simulink library "usask_tlm_lib"  (R2017b)
settings: Solver=ode45  StartTime=0.0  StopTime=10.0  RelTol=1e-3
undefined symbols (not defined in the file or in its folder): B, beta, d, K, L, lambda_1, m_E, m_G, mE_1, mE_2, mG_1, mG_2, nu, r1, r2, rho, T, Zc, Zc_1, Zc_2
libraries: usask_tlm_lib x6, transmission_lines x2
(part 3 of 4)

== system usask_tlm_lib/Elastic TLM Q1P2/G_1 ==
  note: Equation (17) from ven der Buhs et al. 2017
  F + P_1 : Inport
  Sum : Sum  Inputs=+------
  k = 1 : TransferFcn  Numerator=[m_G(1)*T 0]  Denominator=[T n(1)]
  k = 2 : TransferFcn  Numerator=[m_G(2)*T 0]  Denominator=[T n(2)]
  k = 3 : TransferFcn  Numerator=[m_G(3)*T 0]  Denominator=[T n(3)]
  k = 4 : TransferFcn  Numerator=[m_G(4)*T 0]  Denominator=[T n(4)]
  k = 5 : TransferFcn  Numerator=[m_G(5)*T 0]  Denominator=[T n(5)]
  k = 6 : TransferFcn  Numerator=[m_G(6)*T 0]  Denominator=[T n(6)]
  G : Outport
  wires:
  Sum/1 -> G/1
  F + P_1/1 -> k = 4/1, k = 6/1, k = 5/1, k = 1/1, Sum/1, k = 2/1, k = 3/1
  k = 3/1 -> Sum/4
  k = 1/1 -> Sum/2
  k = 2/1 -> Sum/3
  k = 4/1 -> Sum/5
  k = 5/1 -> Sum/6
  k = 6/1 -> Sum/7

== system usask_tlm_lib/Elastic TLM Q1P2/G_2 ==
  note: Equation (17) from ven der Buhs et al. 2017
  F + P_2 : Inport
  Sum : Sum  Inputs=+------
  k = 1 : TransferFcn  Numerator=[m_G(1)*T 0]  Denominator=[T n(1)]
  k = 2 : TransferFcn  Numerator=[m_G(2)*T 0]  Denominator=[T n(2)]
  k = 3 : TransferFcn  Numerator=[m_G(3)*T 0]  Denominator=[T n(3)]
  k = 4 : TransferFcn  Numerator=[m_G(4)*T 0]  Denominator=[T n(4)]
  k = 5 : TransferFcn  Numerator=[m_G(5)*T 0]  Denominator=[T n(5)]
  k = 6 : TransferFcn  Numerator=[m_G(6)*T 0]  Denominator=[T n(6)]
  G : Outport
  wires:
  Sum/1 -> G/1
  F + P_2/1 -> k = 4/1, k = 6/1, k = 5/1, k = 1/1, Sum/1, k = 2/1, k = 3/1
  k = 3/1 -> Sum/4
  k = 1/1 -> Sum/2
  k = 2/1 -> Sum/3
  k = 4/1 -> Sum/5
  k = 5/1 -> Sum/6
  k = 6/1 -> Sum/7

== system usask_tlm_lib/Elastic TLM Q1Q2/  Delay_2  ==
  G : Inport
  Transport Delay : TransportDelay  DelayTime=T_prime
  delay : Outport
  wires:
  G/1 -> Transport Delay/1
  Transport Delay/1 -> delay/1

== system usask_tlm_lib/Elastic TLM Q1Q2/Delay_1  ==
  G : Inport
  Transport Delay : TransportDelay  DelayTime=T_prime
  delay : Outport
  wires:
  G/1 -> Transport Delay/1
  Transport Delay/1 -> delay/1

== system usask_tlm_lib/Elastic TLM Q1Q2/E_1 ==
  note: Equation (14) from ven der Buhs et al. 2017
  Q_1 : Inport
  Gain : Gain  Gain=Z_c
  Sum : Sum  Inputs=++++++
  k = 1 : TransferFcn  Numerator=[m_E(1)]  Denominator=[T n(1)]
  k = 2 : TransferFcn  Numerator=[m_E(2)]  Denominator=[T n(2)]
  k = 3 : TransferFcn  Numerator=[m_E(3)]  Denominator=[T n(3)]
  k = 4 : TransferFcn  Numerator=[m_E(4)]  Denominator=[T n(4)]
  k = 5 : TransferFcn  Numerator=[m_E(5)]  Denominator=[T n(5)]
  k = 6 : TransferFcn  Numerator=[m_E(6)]  Denominator=[T n(6)]
  E : Outport
  wires:
  Gain/1 -> E/1
  Sum/1 -> Gain/1
  k = 1/1 -> Sum/1
  k = 2/1 -> Sum/2
  k = 3/1 -> Sum/3
  k = 4/1 -> Sum/4
  k = 5/1 -> Sum/5
  k = 6/1 -> Sum/6
  Q_1/1 -> k = 2/1, k = 1/1, k = 3/1, k = 6/1, k = 5/1, k = 4/1

== system usask_tlm_lib/Elastic TLM Q1Q2/E_2 ==
  note: Equation (14) from ven der Buhs et al. 2017
  Q_2 : Inport
  Gain : Gain  Gain=Z_c
  Sum : Sum  Inputs=++++++
  k = 1 : TransferFcn  Numerator=[m_E(1)]  Denominator=[T n(1)]
  k = 2 : TransferFcn  Numerator=[m_E(2)]  Denominator=[T n(2)]
  k = 3 : TransferFcn  Numerator=[m_E(3)]  Denominator=[T n(3)]
  k = 4 : TransferFcn  Numerator=[m_E(4)]  Denominator=[T n(4)]
  k = 5 : TransferFcn  Numerator=[m_E(5)]  Denominator=[T n(5)]
  k = 6 : TransferFcn  Numerator=[m_E(6)]  Denominator=[T n(6)]
  E : Outport
  wires:
  Gain/1 -> E/1
  Sum/1 -> Gain/1
  k = 1/1 -> Sum/1
  k = 2/1 -> Sum/2
  k = 3/1 -> Sum/3
  k = 4/1 -> Sum/4
  k = 5/1 -> Sum/5
  k = 6/1 -> Sum/6
  Q_2/1 -> k = 2/1, k = 1/1, k = 3/1, k = 6/1, k = 5/1, k = 4/1

== system usask_tlm_lib/Elastic TLM Q1Q2/F_1 ==
  note: Equation (15) from ven der Buhs et al. 2017
  Q_1 : Inport
  E : Inport  Port=2
  Gain : Gain  Gain=b
  Gain1 : Gain  Gain=Z_c
  Sum : Sum
  F : Outport
  wires:
  Gain/1 -> Sum/2
  Gain1/1 -> Sum/1
  Sum/1 -> F/1
  Q_1/1 -> Gain1/1
  E/1 -> Gain/1

== system usask_tlm_lib/Elastic TLM Q1Q2/F_2 ==
  note: Equation (15) from ven der Buhs et al. 2017
  E : Inport
  Q_2 : Inport  Port=2
  Gain : Gain  Gain=b
  Gain1 : Gain  Gain=Z_c
  Sum : Sum
  F : Outport
  wires:
  E/1 -> Gain/1
  Q_2/1 -> Gain1/1
  Sum/1 -> F/1
  Gain1/1 -> Sum/1
  Gain/1 -> Sum/2

== system usask_tlm_lib/Elastic TLM Q1Q2/G_1 ==
  note: Equation (17) from ven der Buhs et al. 2017
  F + P_1 : Inport
  Sum : Sum  Inputs=+------
  k = 1 : TransferFcn  Numerator=[m_G(1)*T 0]  Denominator=[T n(1)]
  k = 2 : TransferFcn  Numerator=[m_G(2)*T 0]  Denominator=[T n(2)]
  k = 3 : TransferFcn  Numerator=[m_G(3)*T 0]  Denominator=[T n(3)]
  k = 4 : TransferFcn  Numerator=[m_G(4)*T 0]  Denominator=[T n(4)]
  k = 5 : TransferFcn  Numerator=[m_G(5)*T 0]  Denominator=[T n(5)]
  k = 6 : TransferFcn  Numerator=[m_G(6)*T 0]  Denominator=[T n(6)]
  G : Outport
  wires:
  Sum/1 -> G/1
  F + P_1/1 -> k = 4/1, k = 6/1, k = 5/1, k = 1/1, Sum/1, k = 2/1, k = 3/1
  k = 3/1 -> Sum/4
  k = 1/1 -> Sum/2
  k = 2/1 -> Sum/3
  k = 4/1 -> Sum/5
  k = 5/1 -> Sum/6
  k = 6/1 -> Sum/7

== system usask_tlm_lib/Elastic TLM Q1Q2/G_2 ==
  note: Equation (17) from ven der Buhs et al. 2017
  F + P_2 : Inport
  Sum : Sum  Inputs=+------
  k = 1 : TransferFcn  Numerator=[m_G(1)*T 0]  Denominator=[T n(1)]
  k = 2 : TransferFcn  Numerator=[m_G(2)*T 0]  Denominator=[T n(2)]
  k = 3 : TransferFcn  Numerator=[m_G(3)*T 0]  Denominator=[T n(3)]
  k = 4 : TransferFcn  Numerator=[m_G(4)*T 0]  Denominator=[T n(4)]
  k = 5 : TransferFcn  Numerator=[m_G(5)*T 0]  Denominator=[T n(5)]
  k = 6 : TransferFcn  Numerator=[m_G(6)*T 0]  Denominator=[T n(6)]
  G : Outport
  wires:
  Sum/1 -> G/1
  F + P_2/1 -> k = 4/1, k = 6/1, k = 5/1, k = 1/1, Sum/1, k = 2/1, k = 3/1
  k = 3/1 -> Sum/4
  k = 1/1 -> Sum/2
  k = 2/1 -> Sum/3
  k = 4/1 -> Sum/5
  k = 5/1 -> Sum/6
  k = 6/1 -> Sum/7

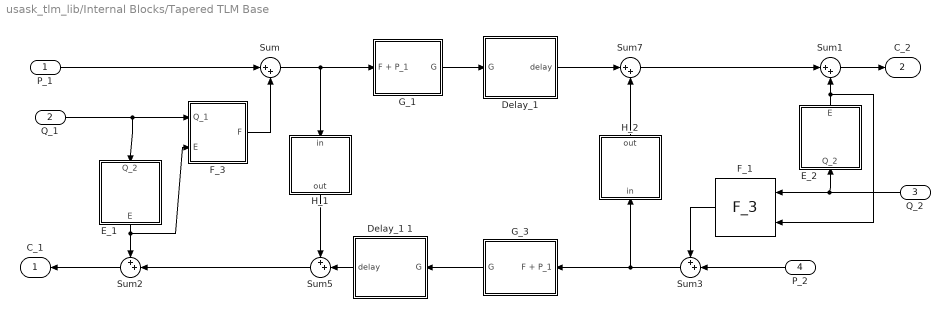
== system usask_tlm_lib/Internal Blocks/Tapered TLM Base ==
  P_1 : Inport
  Q_1 : Inport  Port=2
  Q_2 : Inport  Port=3
  P_2 : Inport  Port=4
  "Delay_1 " : Subsystem  mask{T=T_1}
      mask prompts: T "delay time"
      mask Display: disp('\fontname{Times New Roman}\ite^{-j\omegaT}', 'texmode', 'on')
  Delay_1 1 : Subsystem  mask{T=T_2}
      mask prompts: T "delay time"
      mask Display: disp('\fontname{Times New Roman}\ite^{-j\omegaT}', 'texmode', 'on')
  E_1 : Subsystem  mask{m_E=mE_1, n=n, T=T_1, Zc=Zc_1}
      mask prompts: m_E "mE"
      mask Display: disp('\fontname{Times New Roman}\fontsize{30}\itE', 'texmode', 'on')
  E_2 : Subsystem  mask{m_E=mE_2, n=n, T=T_2, Zc=Zc_2}
      mask prompts: m_E "mE"
      mask Display: disp('\fontname{Times New Roman}\fontsize{30}\itE', 'texmode', 'on')
  F_1 : usask_tlm_lib/Internal Blocks/Tapered TLM Base/F_3  Zc=Zc_2  b=b_2  F_k=F_k2
      settings: SourceProductName=USask Transmission Line Model Library
  F_3 : Subsystem  mask{Zc=Zc_1, b=b_1, F_k=F_k1}
      mask prompts: F_k "Scale"
      mask Display: disp('\fontname{Times New Roman}\fontsize{30}\itF', 'texmode', 'on')
  G_1 : Subsystem  mask{m_G=mG_1, n=n, T=T_1, H_DC=H_2DC}
      mask prompts: m_G "mG"
      mask Display: disp('\fontname{Times New Roman}\fontsize{30}\itG', 'texmode', 'on')
  G_3 : Subsystem  mask{m_G=mG_2, n=n, T=T_2, H_DC=H_1DC}
      mask prompts: m_G "mG"
      mask Display: disp('\fontname{Times New Roman}\fontsize{30}\itG', 'texmode', 'on')
  H_1 : Subsystem  mask{H_a=H_1a, H_b=H_1b, T=T_1+T_2}
      mask prompts: T "T (round trip)"
      mask Display: disp('\fontname{Times New Roman}\fontsize{30}\itH', 'texmode', 'on')
  H_2 : Subsystem  mask{H_a=H_2a, H_b=H_2b, T=T_1+T_2}
      mask prompts: T "T (round trip)"
      mask Display: disp('\fontname{Times New Roman}\fontsize{30}\itH', 'texmode', 'on')
  Sum : Sum  Inputs=|++
  Sum1 : Sum  Inputs=|++
  Sum2 : Sum  Inputs=++|
  Sum3 : Sum  Inputs=++|
  Sum5 : Sum  Inputs=++|
  Sum7 : Sum  Inputs=|++
  C_1 : Outport
  " C_2" : Outport  Port=2
  wires:
  F_1/1 -> Sum3/1
  Sum5/1 -> Sum2/2
  F_3/1(F) -> Sum/2
  P_2/1 -> Sum3/2
  E_2/1(E) -> F_1/2, Sum1/2
  G_1/1(G) -> "Delay_1 "/1(G)
  Q_2/1 -> F_1/1, E_2/1(Q_2)
  Q_1/1 -> F_3/1(Q_1), E_1/1(Q_2)
  Sum1/1 -> " C_2"/1
  Sum3/1 -> G_3/1(F + P_1), H_2/1(in)
  Sum7/1 -> Sum1/1
  H_2/1(out) -> Sum7/2
  Delay_1 1/1(delay) -> Sum5/2
  E_1/1(E) -> F_3/2(E), Sum2/1
  Sum2/1 -> C_1/1
  Sum/1 -> H_1/1(in), G_1/1(F + P_1)
  P_1/1 -> Sum/1
  H_1/1(out) -> Sum5/1
  G_3/1(G) -> Delay_1 1/1(G)
  "Delay_1 "/1(delay) -> Sum7/1

== system usask_tlm_lib/Internal Blocks/Tapered TLM Segment ==
  C_1in : Inport
  C_2in : Inport  Port=2
  Add : Sum
  Add1 : Sum
  Add2 : Sum  Inputs=+-
  Add3 : Sum  Inputs=+-
  Gain{,1..2,4} (4 alike) : Gain  Gain=1/2
  Gain3 : Gain  Gain=1/Zc_1
  Gain5 : Gain  Gain=1/Zc_2
  Tapered TLM Base : usask_tlm_lib/Internal Blocks/Tapered TLM Base  Zc_1=Zc_1  Zc_2=Zc_2  beta=beta  T=T  lambda_1=lambda_1
      settings: SourceProductName=USask Transmission Line Model Library
  " C_1out" : Outport
  " C_2out" : Outport  Port=2
  wires:
  C_1in/1 -> Add/2, Add2/1
  Tapered TLM Base/1 -> " C_1out"/1, Add/1, Add2/2
  Add/1 -> Gain/1
  Gain/1 -> Tapered TLM Base/1
  Gain1/1 -> Tapered TLM Base/4
  Add1/1 -> Gain1/1
  Tapered TLM Base/2 -> " C_2out"/1, Add3/2, Add1/2
  Add2/1 -> Gain2/1
  Gain2/1 -> Gain3/1
  Gain3/1 -> Tapered TLM Base/2
  Gain4/1 -> Gain5/1
  Add3/1 -> Gain4/1
  Gain5/1 -> Tapered TLM Base/3
  C_2in/1 -> Add3/1, Add1/1

== system usask_tlm_lib/TLM Johnston P1P2/E2 ==
  In : Inport
  Transfer Fcn : TransferFcn  Numerator=[R]  Denominator=[K*T 1]
  Out : Outport
  wires:
  Transfer Fcn/1 -> Out/1
  In/1 -> Transfer Fcn/1

== system usask_tlm_lib/TLM Johnston P1P2/F2 ==
  In : Inport
  Gain : Gain  Gain=Zc
  Out : Outport
  wires:
  Gain/1 -> Out/1
  In/1 -> Gain/1

== system usask_tlm_lib/TLM Johnston P1P2/G1 ==
  In : Inport
  G2 : Subsystem  mask(Johnston G2){modelNumber=modelNumber}
      mask prompts: modelNumber "Model"
      mask help: This implements Johnston's G2 models. Model may be 1, 2 or 3 (see paper). Model 1 may be unstable for large beta.
      mask init:
      | k=4;%this must match order of diagram
      | m=nan(k,1);
      | m(1)=2.2457;
      | if k>1
      | m(2)=6.8400;
      | end
      | for i=3:k
      |     m(i)=3*m(i-1);
      | end
      | 
      | 
      | n=nan(k,1);
      | n(1)=42.849;
      | for i=2:k
      |     n(i)=9*n(i-1);
      | end
      | 
      | 
      | if modelNumber==1
      |         bypass1=false;
      |         bypass2=true;
      |         numGain=2;%numerator gain
      | elseif modelNumber==2
      |     bypass1=true;
      |         bypass2=false;
      |         numGain=2;%numerator gain
      | elseif modelNumber==3
      |         bypass1=false;
      |         bypass2=false;
      |         numGain=1;%numerator gain
      | else
      |     warning('Model number must be 1, 2, or 3')
      | end
  Transfer Fcn : TransferFcn  Numerator=[K*beta*r^2/nu*exp(-4*beta) 1]  Denominator=[K*beta*r^2/nu 1]
  Out : Outport
  wires:
  In/1 -> Transfer Fcn/1
  Transfer Fcn/1 -> G2/1(In)
  G2/1(Out) -> Out/1

== system usask_tlm_lib/TLM Johnston P1P2/G2 ==
  In : Inport
  G2 : Subsystem  mask(Johnston G2){modelNumber=modelNumber}
      mask prompts: modelNumber "Model"
      mask help: This implements Johnston's G2 models. Model may be 1, 2 or 3 (see paper). Model 1 may be unstable for large beta.
      mask init: same as usask_tlm_lib/TLM Johnston P1P2/G1/G2
  Transfer Fcn : TransferFcn  Numerator=[K*beta*r^2/nu*exp(-4*beta) 1]  Denominator=[K*beta*r^2/nu 1]
  Out : Outport
  wires:
  In/1 -> Transfer Fcn/1
  Transfer Fcn/1 -> G2/1(In)
  G2/1(Out) -> Out/1

== system usask_tlm_lib/TLM Johnston P1Q2/Ea ==
  In : Inport
  Transfer Fcn : TransferFcn  Numerator=[R]  Denominator=[K*T 1]
  Out : Outport
  wires:
  In/1 -> Transfer Fcn/1
  Transfer Fcn/1 -> Out/1

== system usask_tlm_lib/TLM Johnston P1Q2/Eb ==
  In : Inport
  Transfer Fcn : TransferFcn  Numerator=[R]  Denominator=[K*T 1]
  Out : Outport
  wires:
  In/1 -> Transfer Fcn/1
  Transfer Fcn/1 -> Out/1

== system usask_tlm_lib/TLM Johnston P1Q2/Fa ==
  In : Inport
  Gain : Gain  Gain=Zc
  Out : Outport
  wires:
  In/1 -> Gain/1
  Gain/1 -> Out/1

== system usask_tlm_lib/TLM Johnston P1Q2/Fb ==
  In : Inport
  Gain : Gain  Gain=Zc
  Out : Outport
  wires:
  In/1 -> Gain/1
  Gain/1 -> Out/1

== system usask_tlm_lib/TLM Johnston P1Q2/Ga ==
  In : Inport
  G2 : Subsystem  mask(Johnston G2){modelNumber=modelNumber}
      mask prompts: modelNumber "Model"
      mask help: This implements Johnston's G2 models. Model may be 1, 2 or 3 (see paper). Model 1 may be unstable for large beta.
      mask init: same as usask_tlm_lib/TLM Johnston P1P2/G1/G2
  Transfer Fcn : TransferFcn  Numerator=[K*beta*r^2/nu*exp(-4*beta) 1]  Denominator=[K*beta*r^2/nu 1]
  Out : Outport
  wires:
  G2/1(Out) -> Out/1
  Transfer Fcn/1 -> G2/1(In)
  In/1 -> Transfer Fcn/1

== system usask_tlm_lib/TLM Johnston P1Q2/Gb ==
  In : Inport
  G2 : Subsystem  mask(Johnston G2){modelNumber=modelNumber}
      mask prompts: modelNumber "Model"
      mask help: This implements Johnston's G2 models. Model may be 1, 2 or 3 (see paper). Model 1 may be unstable for large beta.
      mask init: same as usask_tlm_lib/TLM Johnston P1P2/G1/G2
  Transfer Fcn : TransferFcn  Numerator=[K*beta*r^2/nu*exp(-4*beta) 1]  Denominator=[K*beta*r^2/nu 1]
  Out : Outport
  wires:
  G2/1(Out) -> Out/1
  Transfer Fcn/1 -> G2/1(In)
  In/1 -> Transfer Fcn/1

== system usask_tlm_lib/TLM Johnston Q1P2/Ea ==
  In : Inport
  Transfer Fcn : TransferFcn  Numerator=[R]  Denominator=[K*T 1]
  Out : Outport
  wires:
  In/1 -> Transfer Fcn/1
  Transfer Fcn/1 -> Out/1

== system usask_tlm_lib/TLM Johnston Q1P2/Eb ==
  In : Inport
  Transfer Fcn : TransferFcn  Numerator=[R]  Denominator=[K*T 1]
  Out : Outport
  wires:
  In/1 -> Transfer Fcn/1
  Transfer Fcn/1 -> Out/1

== system usask_tlm_lib/TLM Johnston Q1P2/Fa ==
  In : Inport
  Gain : Gain  Gain=Zc
  Out : Outport
  wires:
  In/1 -> Gain/1
  Gain/1 -> Out/1

== system usask_tlm_lib/TLM Johnston Q1P2/Fb ==
  In : Inport
  Gain : Gain  Gain=Zc
  Out : Outport
  wires:
  In/1 -> Gain/1
  Gain/1 -> Out/1

== system usask_tlm_lib/TLM Johnston Q1P2/Ga ==
  In : Inport
  G2 : Subsystem  mask(Johnston G2){modelNumber=modelNumber}
      mask prompts: modelNumber "Model"
      mask help: This implements Johnston's G2 models. Model may be 1, 2 or 3 (see paper). Model 1 may be unstable for large beta.
      mask init: same as usask_tlm_lib/TLM Johnston P1P2/G1/G2
  Transfer Fcn : TransferFcn  Numerator=[K*beta*r^2/nu*exp(-4*beta) 1]  Denominator=[K*beta*r^2/nu 1]
  Out : Outport
  wires:
  G2/1(Out) -> Out/1
  Transfer Fcn/1 -> G2/1(In)
  In/1 -> Transfer Fcn/1

== system usask_tlm_lib/TLM Johnston Q1P2/Gb ==
  In : Inport
  G2 : Subsystem  mask(Johnston G2){modelNumber=modelNumber}
      mask prompts: modelNumber "Model"
      mask help: This implements Johnston's G2 models. Model may be 1, 2 or 3 (see paper). Model 1 may be unstable for large beta.
      mask init: same as usask_tlm_lib/TLM Johnston P1P2/G1/G2
  Transfer Fcn : TransferFcn  Numerator=[K*beta*r^2/nu*exp(-4*beta) 1]  Denominator=[K*beta*r^2/nu 1]
  Out : Outport
  wires:
  G2/1(Out) -> Out/1
  Transfer Fcn/1 -> G2/1(In)
  In/1 -> Transfer Fcn/1

== system usask_tlm_lib/TLM Johnston Q1Q2/Ea ==
  In : Inport
  Transfer Fcn : TransferFcn  Numerator=[R]  Denominator=[K*T 1]
  Out : Outport
  wires:
  In/1 -> Transfer Fcn/1
  Transfer Fcn/1 -> Out/1

== system usask_tlm_lib/TLM Johnston Q1Q2/Eb ==
  In : Inport
  Transfer Fcn : TransferFcn  Numerator=[R]  Denominator=[K*T 1]
  Out : Outport
  wires:
  In/1 -> Transfer Fcn/1
  Transfer Fcn/1 -> Out/1

== system usask_tlm_lib/TLM Johnston Q1Q2/Fa ==
  In : Inport
  Gain : Gain  Gain=Zc
  Out : Outport
  wires:
  In/1 -> Gain/1
  Gain/1 -> Out/1

== system usask_tlm_lib/TLM Johnston Q1Q2/Fb ==
  In : Inport
  Gain : Gain  Gain=Zc
  Out : Outport
  wires:
  In/1 -> Gain/1
  Gain/1 -> Out/1

== system usask_tlm_lib/TLM Johnston Q1Q2/Ga ==
  In : Inport
  G2 : Subsystem  mask(Johnston G2){modelNumber=modelNumber}
      mask prompts: modelNumber "Model"
      mask help: This implements Johnston's G2 models. Model may be 1, 2 or 3 (see paper). Model 1 may be unstable for large beta.
      mask init: same as usask_tlm_lib/TLM Johnston P1P2/G1/G2
  Transfer Fcn : TransferFcn  Numerator=[K*beta*r^2/nu*exp(-4*beta) 1]  Denominator=[K*beta*r^2/nu 1]
  Out : Outport
  wires:
  G2/1(Out) -> Out/1
  Transfer Fcn/1 -> G2/1(In)
  In/1 -> Transfer Fcn/1

== system usask_tlm_lib/TLM Johnston Q1Q2/Gb ==
  In : Inport
  G2 : Subsystem  mask(Johnston G2){modelNumber=modelNumber}
      mask prompts: modelNumber "Model"
      mask help: This implements Johnston's G2 models. Model may be 1, 2 or 3 (see paper). Model 1 may be unstable for large beta.
      mask init: same as usask_tlm_lib/TLM Johnston P1P2/G1/G2
  Transfer Fcn : TransferFcn  Numerator=[K*beta*r^2/nu*exp(-4*beta) 1]  Denominator=[K*beta*r^2/nu 1]
  Out : Outport
  wires:
  G2/1(Out) -> Out/1
  Transfer Fcn/1 -> G2/1(In)
  In/1 -> Transfer Fcn/1

== system usask_tlm_lib/TLM Krus P1P2/E1 ==
  In : Inport
  Transfer Fcn : TransferFcn  Numerator=[R]  Denominator=[K*T 1]
  Out : Outport
  wires:
  Transfer Fcn/1 -> Out/1
  In/1 -> Transfer Fcn/1

== system usask_tlm_lib/TLM Krus P1P2/E2 ==
  In : Inport
  Transfer Fcn : TransferFcn  Numerator=[R]  Denominator=[K*T 1]
  Out : Outport
  wires:
  Transfer Fcn/1 -> Out/1
  In/1 -> Transfer Fcn/1

== system usask_tlm_lib/TLM Krus P1P2/F1 ==
  In : Inport
  Gain : Gain  Gain=Zc
  Out : Outport
  wires:
  Gain/1 -> Out/1
  In/1 -> Gain/1

== system usask_tlm_lib/TLM Krus P1P2/F2 ==
  In : Inport
  Gain : Gain  Gain=Zc
  Out : Outport
  wires:
  Gain/1 -> Out/1
  In/1 -> Gain/1

== system usask_tlm_lib/TLM Krus P1P2/G1 ==
  In : Inport
  Transfer Fcn : TransferFcn  Numerator=[K*T*exp(-R*A/(2*rho*c)) 1]  Denominator=[K*T 1]
  Out : Outport
  wires:
  Transfer Fcn/1 -> Out/1
  In/1 -> Transfer Fcn/1

== system usask_tlm_lib/TLM Krus P1P2/G2 ==
  In : Inport
  Transfer Fcn : TransferFcn  Numerator=[K*T*exp(-R*A/(2*rho*c)) 1]  Denominator=[K*T 1]
  Out : Outport
  wires:
  Transfer Fcn/1 -> Out/1
  In/1 -> Transfer Fcn/1

== system usask_tlm_lib/TLM Krus P1Q2/E1 ==
  In : Inport
  Transfer Fcn : TransferFcn  Numerator=[R]  Denominator=[K*T 1]
  Out : Outport
  wires:
  In/1 -> Transfer Fcn/1
  Transfer Fcn/1 -> Out/1

== system usask_tlm_lib/TLM Krus P1Q2/E2 ==
  In : Inport
  Transfer Fcn : TransferFcn  Numerator=[R]  Denominator=[K*T 1]
  Out : Outport
  wires:
  In/1 -> Transfer Fcn/1
  Transfer Fcn/1 -> Out/1

== system usask_tlm_lib/TLM Krus P1Q2/F1 ==
  In : Inport
  Gain : Gain  Gain=Zc
  Out : Outport
  wires:
  In/1 -> Gain/1
  Gain/1 -> Out/1

== system usask_tlm_lib/TLM Krus P1Q2/F2 ==
  In : Inport
  Gain : Gain  Gain=Zc
  Out : Outport
  wires:
  In/1 -> Gain/1
  Gain/1 -> Out/1

== system usask_tlm_lib/TLM Krus P1Q2/G1 ==
  In : Inport
  Transfer Fcn : TransferFcn  Numerator=[K*T*exp(-R*A/(2*rho*c)) 1]  Denominator=[K*T 1]
  Out : Outport
  wires:
  In/1 -> Transfer Fcn/1
  Transfer Fcn/1 -> Out/1

== system usask_tlm_lib/TLM Krus P1Q2/G2 ==
  In : Inport
  Transfer Fcn : TransferFcn  Numerator=[K*T*exp(-R*A/(2*rho*c)) 1]  Denominator=[K*T 1]
  Out : Outport
  wires:
  In/1 -> Transfer Fcn/1
  Transfer Fcn/1 -> Out/1

== system usask_tlm_lib/TLM Krus Q1P2/E1 ==
  In : Inport
  Transfer Fcn : TransferFcn  Numerator=[R]  Denominator=[K*T 1]
  Out : Outport
  wires:
  Transfer Fcn/1 -> Out/1
  In/1 -> Transfer Fcn/1

== system usask_tlm_lib/TLM Krus Q1P2/E2 ==
  In : Inport
  Transfer Fcn : TransferFcn  Numerator=[R]  Denominator=[K*T 1]
  Out : Outport
  wires:
  Transfer Fcn/1 -> Out/1
  In/1 -> Transfer Fcn/1

== system usask_tlm_lib/TLM Krus Q1P2/F1 ==
  In : Inport
  Gain : Gain  Gain=Zc
  Out : Outport
  wires:
  Gain/1 -> Out/1
  In/1 -> Gain/1

== system usask_tlm_lib/TLM Krus Q1P2/F2 ==
  In : Inport
  Gain : Gain  Gain=Zc
  Out : Outport
  wires:
  Gain/1 -> Out/1
  In/1 -> Gain/1

== system usask_tlm_lib/TLM Krus Q1P2/G1 ==
  In : Inport
  Transfer Fcn : TransferFcn  Numerator=[K*T*exp(-R*A/(2*rho*c)) 1]  Denominator=[K*T 1]
  Out : Outport
  wires:
  Transfer Fcn/1 -> Out/1
  In/1 -> Transfer Fcn/1

== system usask_tlm_lib/TLM Krus Q1P2/G2 ==
  In : Inport
  Transfer Fcn : TransferFcn  Numerator=[K*T*exp(-R*A/(2*rho*c)) 1]  Denominator=[K*T 1]
  Out : Outport
  wires:
  Transfer Fcn/1 -> Out/1
  In/1 -> Transfer Fcn/1

== system usask_tlm_lib/TLM Krus Q1Q2/E1 ==
  In : Inport
  Transfer Fcn : TransferFcn  Numerator=[R]  Denominator=[K*T 1]
  Out : Outport
  wires:
  Transfer Fcn/1 -> Out/1
  In/1 -> Transfer Fcn/1

== system usask_tlm_lib/TLM Krus Q1Q2/E2 ==
  In : Inport
  Transfer Fcn : TransferFcn  Numerator=[R]  Denominator=[K*T 1]
  Out : Outport
  wires:
  Transfer Fcn/1 -> Out/1
  In/1 -> Transfer Fcn/1

== system usask_tlm_lib/TLM Krus Q1Q2/F1 ==
  In : Inport
  Gain : Gain  Gain=Zc
  Out : Outport
  wires:
  Gain/1 -> Out/1
  In/1 -> Gain/1

== system usask_tlm_lib/TLM Krus Q1Q2/F2 ==
  In : Inport
  Gain : Gain  Gain=Zc
  Out : Outport
  wires:
  Gain/1 -> Out/1
  In/1 -> Gain/1

== system usask_tlm_lib/TLM Krus Q1Q2/G1 ==
  In : Inport
  Transfer Fcn : TransferFcn  Numerator=[K*T*exp(-R*A/(2*rho*c)) 1]  Denominator=[K*T 1]
  Out : Outport
  wires:
  Transfer Fcn/1 -> Out/1
  In/1 -> Transfer Fcn/1

== system usask_tlm_lib/TLM Krus Q1Q2/G2 ==
  In : Inport
  Transfer Fcn : TransferFcn  Numerator=[K*T*exp(-R*A/(2*rho*c)) 1]  Denominator=[K*T 1]
  Out : Outport
  wires:
  Transfer Fcn/1 -> Out/1
  In/1 -> Transfer Fcn/1

== system usask_tlm_lib/Tapered Elastic TLM P1P2/  Delay_2  ==
  G : Inport
  Transport Delay : TransportDelay  DelayTime=T_prime
  delay : Outport
  wires:
  G/1 -> Transport Delay/1
  Transport Delay/1 -> delay/1

== system usask_tlm_lib/Tapered Elastic TLM P1P2/Delay_1  ==
  G : Inport
  Transport Delay : TransportDelay  DelayTime=T_prime
  delay : Outport
  wires:
  G/1 -> Transport Delay/1
  Transport Delay/1 -> delay/1

== system usask_tlm_lib/Tapered Elastic TLM P1P2/E_1 ==
  note: Equation (14) from ven der Buhs et al. 2017
  Q_1 : Inport
  Gain : Gain  Gain=Z_c
  Sum : Sum  Inputs=++++++
  k = 1 : TransferFcn  Numerator=[m_E(1)]  Denominator=[T n(1)]
  k = 2 : TransferFcn  Numerator=[m_E(2)]  Denominator=[T n(2)]
  k = 3 : TransferFcn  Numerator=[m_E(3)]  Denominator=[T n(3)]
  k = 4 : TransferFcn  Numerator=[m_E(4)]  Denominator=[T n(4)]
  k = 5 : TransferFcn  Numerator=[m_E(5)]  Denominator=[T n(5)]
  k = 6 : TransferFcn  Numerator=[m_E(6)]  Denominator=[T n(6)]
  E : Outport
  wires:
  Gain/1 -> E/1
  Sum/1 -> Gain/1
  k = 1/1 -> Sum/1
  k = 2/1 -> Sum/2
  k = 3/1 -> Sum/3
  k = 4/1 -> Sum/4
  k = 5/1 -> Sum/5
  k = 6/1 -> Sum/6
  Q_1/1 -> k = 2/1, k = 1/1, k = 3/1, k = 6/1, k = 5/1, k = 4/1

== system usask_tlm_lib/Tapered Elastic TLM P1P2/E_2 ==
  note: Equation (14) from ven der Buhs et al. 2017
  Q_2 : Inport
  Gain : Gain  Gain=Z_c
  Sum : Sum  Inputs=++++++
  k = 1 : TransferFcn  Numerator=[m_E(1)]  Denominator=[T n(1)]
  k = 2 : TransferFcn  Numerator=[m_E(2)]  Denominator=[T n(2)]
  k = 3 : TransferFcn  Numerator=[m_E(3)]  Denominator=[T n(3)]
  k = 4 : TransferFcn  Numerator=[m_E(4)]  Denominator=[T n(4)]
  k = 5 : TransferFcn  Numerator=[m_E(5)]  Denominator=[T n(5)]
  k = 6 : TransferFcn  Numerator=[m_E(6)]  Denominator=[T n(6)]
  E : Outport
  wires:
  Gain/1 -> E/1
  Sum/1 -> Gain/1
  k = 1/1 -> Sum/1
  k = 2/1 -> Sum/2
  k = 3/1 -> Sum/3
  k = 4/1 -> Sum/4
  k = 5/1 -> Sum/5
  k = 6/1 -> Sum/6
  Q_2/1 -> k = 2/1, k = 1/1, k = 3/1, k = 6/1, k = 5/1, k = 4/1

== system usask_tlm_lib/Tapered Elastic TLM P1P2/F_1 ==
  note: Equation (15) from ven der Buhs et al. 2017
  Q_1 : Inport
  E : Inport  Port=2
  Gain : Gain  Gain=b
  Gain1 : Gain  Gain=Z_c
  Sum : Sum
  Out1 : Outport
  wires:
  Gain/1 -> Sum/2
  Gain1/1 -> Sum/1
  Sum/1 -> Out1/1
  Q_1/1 -> Gain1/1
  E/1 -> Gain/1

== system usask_tlm_lib/Tapered Elastic TLM P1P2/F_2 ==
  note: Equation (15) from ven der Buhs et al. 2017
  E : Inport
  Q_2 : Inport  Port=2
  Gain : Gain  Gain=b
  Gain1 : Gain  Gain=Z_c
  Sum : Sum
  F : Outport
  wires:
  E/1 -> Gain/1
  Q_2/1 -> Gain1/1
  Sum/1 -> F/1
  Gain1/1 -> Sum/1
  Gain/1 -> Sum/2

== system usask_tlm_lib/Tapered Elastic TLM P1P2/G_1 ==
  note: Equation (17) from ven der Buhs et al. 2017
  F + P_1 : Inport
  Sum : Sum  Inputs=+------
  k = 1 : TransferFcn  Numerator=[m_G(1)*T 0]  Denominator=[T n(1)]
  k = 2 : TransferFcn  Numerator=[m_G(2)*T 0]  Denominator=[T n(2)]
  k = 3 : TransferFcn  Numerator=[m_G(3)*T 0]  Denominator=[T n(3)]
  k = 4 : TransferFcn  Numerator=[m_G(4)*T 0]  Denominator=[T n(4)]
  k = 5 : TransferFcn  Numerator=[m_G(5)*T 0]  Denominator=[T n(5)]
  k = 6 : TransferFcn  Numerator=[m_G(6)*T 0]  Denominator=[T n(6)]
  G : Outport
  wires:
  Sum/1 -> G/1
  F + P_1/1 -> k = 4/1, k = 6/1, k = 5/1, k = 1/1, Sum/1, k = 2/1, k = 3/1
  k = 3/1 -> Sum/4
  k = 1/1 -> Sum/2
  k = 2/1 -> Sum/3
  k = 4/1 -> Sum/5
  k = 5/1 -> Sum/6
  k = 6/1 -> Sum/7

== system usask_tlm_lib/Tapered Elastic TLM P1P2/G_2 ==
  note: Equation (17) from ven der Buhs et al. 2017
  F + P_2 : Inport
  Sum : Sum  Inputs=+------
  k = 1 : TransferFcn  Numerator=[m_G(1)*T 0]  Denominator=[T n(1)]
  k = 2 : TransferFcn  Numerator=[m_G(2)*T 0]  Denominator=[T n(2)]
  k = 3 : TransferFcn  Numerator=[m_G(3)*T 0]  Denominator=[T n(3)]
  k = 4 : TransferFcn  Numerator=[m_G(4)*T 0]  Denominator=[T n(4)]
  k = 5 : TransferFcn  Numerator=[m_G(5)*T 0]  Denominator=[T n(5)]
  k = 6 : TransferFcn  Numerator=[m_G(6)*T 0]  Denominator=[T n(6)]
  G : Outport
  wires:
  Sum/1 -> G/1
  F + P_2/1 -> k = 4/1, k = 6/1, k = 5/1, k = 1/1, Sum/1, k = 2/1, k = 3/1
  k = 3/1 -> Sum/4
  k = 1/1 -> Sum/2
  k = 2/1 -> Sum/3
  k = 4/1 -> Sum/5
  k = 5/1 -> Sum/6
  k = 6/1 -> Sum/7

== system usask_tlm_lib/Tapered Elastic TLM P1Q2/  Delay_2  ==
  G : Inport
  Transport Delay : TransportDelay  DelayTime=T_prime
  delay : Outport
  wires:
  G/1 -> Transport Delay/1
  Transport Delay/1 -> delay/1

== system usask_tlm_lib/Tapered Elastic TLM P1Q2/Delay_1  ==
  G : Inport
  Transport Delay : TransportDelay  DelayTime=T_prime
  delay : Outport
  wires:
  G/1 -> Transport Delay/1
  Transport Delay/1 -> delay/1

== system usask_tlm_lib/Tapered Elastic TLM P1Q2/E_1 ==
  note: Equation (14) from ven der Buhs et al. 2017
  Q_1 : Inport
  Gain : Gain  Gain=Z_c
  Sum : Sum  Inputs=++++++
  k = 1 : TransferFcn  Numerator=[m_E(1)]  Denominator=[T n(1)]
  k = 2 : TransferFcn  Numerator=[m_E(2)]  Denominator=[T n(2)]
  k = 3 : TransferFcn  Numerator=[m_E(3)]  Denominator=[T n(3)]
  k = 4 : TransferFcn  Numerator=[m_E(4)]  Denominator=[T n(4)]
  k = 5 : TransferFcn  Numerator=[m_E(5)]  Denominator=[T n(5)]
  k = 6 : TransferFcn  Numerator=[m_E(6)]  Denominator=[T n(6)]
  E : Outport
  wires:
  Gain/1 -> E/1
  Sum/1 -> Gain/1
  k = 1/1 -> Sum/1
  k = 2/1 -> Sum/2
  k = 3/1 -> Sum/3
  k = 4/1 -> Sum/4
  k = 5/1 -> Sum/5
  k = 6/1 -> Sum/6
  Q_1/1 -> k = 2/1, k = 1/1, k = 3/1, k = 6/1, k = 5/1, k = 4/1

== system usask_tlm_lib/Tapered Elastic TLM P1Q2/E_2 ==
  note: Equation (14) from ven der Buhs et al. 2017
  Q_2 : Inport
  Gain : Gain  Gain=Z_c
  Sum : Sum  Inputs=++++++
  k = 1 : TransferFcn  Numerator=[m_E(1)]  Denominator=[T n(1)]
  k = 2 : TransferFcn  Numerator=[m_E(2)]  Denominator=[T n(2)]
  k = 3 : TransferFcn  Numerator=[m_E(3)]  Denominator=[T n(3)]
  k = 4 : TransferFcn  Numerator=[m_E(4)]  Denominator=[T n(4)]
  k = 5 : TransferFcn  Numerator=[m_E(5)]  Denominator=[T n(5)]
  k = 6 : TransferFcn  Numerator=[m_E(6)]  Denominator=[T n(6)]
  E : Outport
  wires:
  Gain/1 -> E/1
  Sum/1 -> Gain/1
  k = 1/1 -> Sum/1
  k = 2/1 -> Sum/2
  k = 3/1 -> Sum/3
  k = 4/1 -> Sum/4
  k = 5/1 -> Sum/5
  k = 6/1 -> Sum/6
  Q_2/1 -> k = 2/1, k = 1/1, k = 3/1, k = 6/1, k = 5/1, k = 4/1

== system usask_tlm_lib/Tapered Elastic TLM P1Q2/F_1 ==
  note: Equation (15) from ven der Buhs et al. 2017
  Q_1 : Inport
  E : Inport  Port=2
  Gain : Gain  Gain=b
  Gain1 : Gain  Gain=Z_c
  Sum : Sum
  F : Outport
  wires:
  Gain/1 -> Sum/2
  Gain1/1 -> Sum/1
  Sum/1 -> F/1
  Q_1/1 -> Gain1/1
  E/1 -> Gain/1

== system usask_tlm_lib/Tapered Elastic TLM P1Q2/F_2 ==
  note: Equation (15) from ven der Buhs et al. 2017
  E : Inport
  Q_2 : Inport  Port=2
  Gain : Gain  Gain=b
  Gain1 : Gain  Gain=Z_c
  Sum : Sum
  Out1 : Outport
  wires:
  E/1 -> Gain/1
  Q_2/1 -> Gain1/1
  Sum/1 -> Out1/1
  Gain1/1 -> Sum/1
  Gain/1 -> Sum/2

== system usask_tlm_lib/Tapered Elastic TLM P1Q2/G_1 ==
  note: Equation (17) from ven der Buhs et al. 2017
  F + P_1 : Inport
  Sum : Sum  Inputs=+------
  k = 1 : TransferFcn  Numerator=[m_G(1)*T 0]  Denominator=[T n(1)]
  k = 2 : TransferFcn  Numerator=[m_G(2)*T 0]  Denominator=[T n(2)]
  k = 3 : TransferFcn  Numerator=[m_G(3)*T 0]  Denominator=[T n(3)]
  k = 4 : TransferFcn  Numerator=[m_G(4)*T 0]  Denominator=[T n(4)]
  k = 5 : TransferFcn  Numerator=[m_G(5)*T 0]  Denominator=[T n(5)]
  k = 6 : TransferFcn  Numerator=[m_G(6)*T 0]  Denominator=[T n(6)]
  G : Outport
  wires:
  Sum/1 -> G/1
  F + P_1/1 -> k = 4/1, k = 6/1, k = 5/1, k = 1/1, Sum/1, k = 2/1, k = 3/1
  k = 3/1 -> Sum/4
  k = 1/1 -> Sum/2
  k = 2/1 -> Sum/3
  k = 4/1 -> Sum/5
  k = 5/1 -> Sum/6
  k = 6/1 -> Sum/7

== system usask_tlm_lib/Tapered Elastic TLM P1Q2/G_2 ==
  note: Equation (17) from ven der Buhs et al. 2017
  F + P_2 : Inport
  Sum : Sum  Inputs=+------
  k = 1 : TransferFcn  Numerator=[m_G(1)*T 0]  Denominator=[T n(1)]
  k = 2 : TransferFcn  Numerator=[m_G(2)*T 0]  Denominator=[T n(2)]
  k = 3 : TransferFcn  Numerator=[m_G(3)*T 0]  Denominator=[T n(3)]
  k = 4 : TransferFcn  Numerator=[m_G(4)*T 0]  Denominator=[T n(4)]
  k = 5 : TransferFcn  Numerator=[m_G(5)*T 0]  Denominator=[T n(5)]
  k = 6 : TransferFcn  Numerator=[m_G(6)*T 0]  Denominator=[T n(6)]
  G : Outport
  wires:
  Sum/1 -> G/1
  F + P_2/1 -> k = 4/1, k = 6/1, k = 5/1, k = 1/1, Sum/1, k = 2/1, k = 3/1
  k = 3/1 -> Sum/4
  k = 1/1 -> Sum/2
  k = 2/1 -> Sum/3
  k = 4/1 -> Sum/5
  k = 5/1 -> Sum/6
  k = 6/1 -> Sum/7

== system usask_tlm_lib/Tapered Elastic TLM Q1P2/  Delay_2  ==
  G : Inport
  Transport Delay : TransportDelay  DelayTime=T_prime
  delay : Outport
  wires:
  G/1 -> Transport Delay/1
  Transport Delay/1 -> delay/1

== system usask_tlm_lib/Tapered Elastic TLM Q1P2/Delay_1  ==
  G : Inport
  Transport Delay : TransportDelay  DelayTime=T_prime
  delay : Outport
  wires:
  G/1 -> Transport Delay/1
  Transport Delay/1 -> delay/1

== system usask_tlm_lib/Tapered Elastic TLM Q1P2/E_1 ==
  note: Equation (14) from ven der Buhs et al. 2017
  Q_1 : Inport
  Gain : Gain  Gain=Z_c
  Sum : Sum  Inputs=++++++
  k = 1 : TransferFcn  Numerator=[m_E(1)]  Denominator=[T n(1)]
  k = 2 : TransferFcn  Numerator=[m_E(2)]  Denominator=[T n(2)]
  k = 3 : TransferFcn  Numerator=[m_E(3)]  Denominator=[T n(3)]
  k = 4 : TransferFcn  Numerator=[m_E(4)]  Denominator=[T n(4)]
  k = 5 : TransferFcn  Numerator=[m_E(5)]  Denominator=[T n(5)]
  k = 6 : TransferFcn  Numerator=[m_E(6)]  Denominator=[T n(6)]
  E : Outport
  wires:
  Gain/1 -> E/1
  Sum/1 -> Gain/1
  k = 1/1 -> Sum/1
  k = 2/1 -> Sum/2
  k = 3/1 -> Sum/3
  k = 4/1 -> Sum/4
  k = 5/1 -> Sum/5
  k = 6/1 -> Sum/6
  Q_1/1 -> k = 2/1, k = 1/1, k = 3/1, k = 6/1, k = 5/1, k = 4/1

== system usask_tlm_lib/Tapered Elastic TLM Q1P2/E_2 ==
  note: Equation (14) from ven der Buhs et al. 2017
  Q_2 : Inport
  Gain : Gain  Gain=Z_c
  Sum : Sum  Inputs=++++++
  k = 1 : TransferFcn  Numerator=[m_E(1)]  Denominator=[T n(1)]
  k = 2 : TransferFcn  Numerator=[m_E(2)]  Denominator=[T n(2)]
  k = 3 : TransferFcn  Numerator=[m_E(3)]  Denominator=[T n(3)]
  k = 4 : TransferFcn  Numerator=[m_E(4)]  Denominator=[T n(4)]
  k = 5 : TransferFcn  Numerator=[m_E(5)]  Denominator=[T n(5)]
  k = 6 : TransferFcn  Numerator=[m_E(6)]  Denominator=[T n(6)]
  E : Outport
  wires:
  Gain/1 -> E/1
  Sum/1 -> Gain/1
  k = 1/1 -> Sum/1
  k = 2/1 -> Sum/2
  k = 3/1 -> Sum/3
  k = 4/1 -> Sum/4
  k = 5/1 -> Sum/5
  k = 6/1 -> Sum/6
  Q_2/1 -> k = 2/1, k = 1/1, k = 3/1, k = 6/1, k = 5/1, k = 4/1

== system usask_tlm_lib/Tapered Elastic TLM Q1P2/F_1 ==
  note: Equation (15) from ven der Buhs et al. 2017
  Q_1 : Inport
  E : Inport  Port=2
  Gain : Gain  Gain=b
  Gain1 : Gain  Gain=Z_c
  Sum : Sum
  F : Outport
  wires:
  Gain/1 -> Sum/2
  Gain1/1 -> Sum/1
  Sum/1 -> F/1
  Q_1/1 -> Gain1/1
  E/1 -> Gain/1

== system usask_tlm_lib/Tapered Elastic TLM Q1P2/F_2 ==
  note: Equation (15) from ven der Buhs et al. 2017
  E : Inport
  Q_2 : Inport  Port=2
  Gain : Gain  Gain=b
  Gain1 : Gain  Gain=Z_c
  Sum : Sum
  Out1 : Outport
  wires:
  E/1 -> Gain/1
  Q_2/1 -> Gain1/1
  Sum/1 -> Out1/1
  Gain1/1 -> Sum/1
  Gain/1 -> Sum/2

== system usask_tlm_lib/Tapered Elastic TLM Q1P2/G_1 ==
  note: Equation (17) from ven der Buhs et al. 2017
  F + P_1 : Inport
  Sum : Sum  Inputs=+------
  k = 1 : TransferFcn  Numerator=[m_G(1)*T 0]  Denominator=[T n(1)]
  k = 2 : TransferFcn  Numerator=[m_G(2)*T 0]  Denominator=[T n(2)]
  k = 3 : TransferFcn  Numerator=[m_G(3)*T 0]  Denominator=[T n(3)]
  k = 4 : TransferFcn  Numerator=[m_G(4)*T 0]  Denominator=[T n(4)]
  k = 5 : TransferFcn  Numerator=[m_G(5)*T 0]  Denominator=[T n(5)]
  k = 6 : TransferFcn  Numerator=[m_G(6)*T 0]  Denominator=[T n(6)]
  G : Outport
  wires:
  Sum/1 -> G/1
  F + P_1/1 -> k = 4/1, k = 6/1, k = 5/1, k = 1/1, Sum/1, k = 2/1, k = 3/1
  k = 3/1 -> Sum/4
  k = 1/1 -> Sum/2
  k = 2/1 -> Sum/3
  k = 4/1 -> Sum/5
  k = 5/1 -> Sum/6
  k = 6/1 -> Sum/7

== system usask_tlm_lib/Tapered Elastic TLM Q1P2/G_2 ==
  note: Equation (17) from ven der Buhs et al. 2017
  F + P_2 : Inport
  Sum : Sum  Inputs=+------
  k = 1 : TransferFcn  Numerator=[m_G(1)*T 0]  Denominator=[T n(1)]
  k = 2 : TransferFcn  Numerator=[m_G(2)*T 0]  Denominator=[T n(2)]
  k = 3 : TransferFcn  Numerator=[m_G(3)*T 0]  Denominator=[T n(3)]
  k = 4 : TransferFcn  Numerator=[m_G(4)*T 0]  Denominator=[T n(4)]
  k = 5 : TransferFcn  Numerator=[m_G(5)*T 0]  Denominator=[T n(5)]
  k = 6 : TransferFcn  Numerator=[m_G(6)*T 0]  Denominator=[T n(6)]
  G : Outport
  wires:
  Sum/1 -> G/1
  F + P_2/1 -> k = 4/1, k = 6/1, k = 5/1, k = 1/1, Sum/1, k = 2/1, k = 3/1
  k = 3/1 -> Sum/4
  k = 1/1 -> Sum/2
  k = 2/1 -> Sum/3
  k = 4/1 -> Sum/5
  k = 5/1 -> Sum/6
  k = 6/1 -> Sum/7

== system usask_tlm_lib/Tapered Elastic TLM Q1Q2/  Delay_2  ==
  G : Inport
  Transport Delay : TransportDelay  DelayTime=T_prime
  delay : Outport
  wires:
  G/1 -> Transport Delay/1
  Transport Delay/1 -> delay/1

== system usask_tlm_lib/Tapered Elastic TLM Q1Q2/Delay_1  ==
  G : Inport
  Transport Delay : TransportDelay  DelayTime=T_prime
  delay : Outport
  wires:
  G/1 -> Transport Delay/1
  Transport Delay/1 -> delay/1

== system usask_tlm_lib/Tapered Elastic TLM Q1Q2/E_1 ==
  note: Equation (14) from ven der Buhs et al. 2017
  Q_1 : Inport
  Gain : Gain  Gain=Z_c
  Sum : Sum  Inputs=++++++
  k = 1 : TransferFcn  Numerator=[m_E(1)]  Denominator=[T n(1)]
  k = 2 : TransferFcn  Numerator=[m_E(2)]  Denominator=[T n(2)]
  k = 3 : TransferFcn  Numerator=[m_E(3)]  Denominator=[T n(3)]
  k = 4 : TransferFcn  Numerator=[m_E(4)]  Denominator=[T n(4)]
  k = 5 : TransferFcn  Numerator=[m_E(5)]  Denominator=[T n(5)]
  k = 6 : TransferFcn  Numerator=[m_E(6)]  Denominator=[T n(6)]
  E : Outport
  wires:
  Gain/1 -> E/1
  Sum/1 -> Gain/1
  k = 1/1 -> Sum/1
  k = 2/1 -> Sum/2
  k = 3/1 -> Sum/3
  k = 4/1 -> Sum/4
  k = 5/1 -> Sum/5
  k = 6/1 -> Sum/6
  Q_1/1 -> k = 2/1, k = 1/1, k = 3/1, k = 6/1, k = 5/1, k = 4/1

== system usask_tlm_lib/Tapered Elastic TLM Q1Q2/E_2 ==
  note: Equation (14) from ven der Buhs et al. 2017
  Q_2 : Inport
  Gain : Gain  Gain=Z_c
  Sum : Sum  Inputs=++++++
  k = 1 : TransferFcn  Numerator=[m_E(1)]  Denominator=[T n(1)]
  k = 2 : TransferFcn  Numerator=[m_E(2)]  Denominator=[T n(2)]
  k = 3 : TransferFcn  Numerator=[m_E(3)]  Denominator=[T n(3)]
  k = 4 : TransferFcn  Numerator=[m_E(4)]  Denominator=[T n(4)]
  k = 5 : TransferFcn  Numerator=[m_E(5)]  Denominator=[T n(5)]
  k = 6 : TransferFcn  Numerator=[m_E(6)]  Denominator=[T n(6)]
  E : Outport
  wires:
  Gain/1 -> E/1
  Sum/1 -> Gain/1
  k = 1/1 -> Sum/1
  k = 2/1 -> Sum/2
  k = 3/1 -> Sum/3
  k = 4/1 -> Sum/4
  k = 5/1 -> Sum/5
  k = 6/1 -> Sum/6
  Q_2/1 -> k = 2/1, k = 1/1, k = 3/1, k = 6/1, k = 5/1, k = 4/1

== system usask_tlm_lib/Tapered Elastic TLM Q1Q2/F_1 ==
  note: Equation (15) from ven der Buhs et al. 2017
  Q_1 : Inport
  E : Inport  Port=2
  Gain : Gain  Gain=b
  Gain1 : Gain  Gain=Z_c
  Sum : Sum
  F : Outport
  wires:
  Gain/1 -> Sum/2
  Gain1/1 -> Sum/1
  Sum/1 -> F/1
  Q_1/1 -> Gain1/1
  E/1 -> Gain/1

== system usask_tlm_lib/Tapered Elastic TLM Q1Q2/F_2 ==
  note: Equation (15) from ven der Buhs et al. 2017
  E : Inport
  Q_2 : Inport  Port=2
  Gain : Gain  Gain=b
  Gain1 : Gain  Gain=Z_c
  Sum : Sum
  F : Outport
  wires:
  E/1 -> Gain/1
  Q_2/1 -> Gain1/1
  Sum/1 -> F/1
  Gain1/1 -> Sum/1
  Gain/1 -> Sum/2

== system usask_tlm_lib/Tapered Elastic TLM Q1Q2/G_1 ==
  note: Equation (17) from ven der Buhs et al. 2017
  F + P_1 : Inport
  Sum : Sum  Inputs=+------
  k = 1 : TransferFcn  Numerator=[m_G(1)*T 0]  Denominator=[T n(1)]
  k = 2 : TransferFcn  Numerator=[m_G(2)*T 0]  Denominator=[T n(2)]
  k = 3 : TransferFcn  Numerator=[m_G(3)*T 0]  Denominator=[T n(3)]
  k = 4 : TransferFcn  Numerator=[m_G(4)*T 0]  Denominator=[T n(4)]
  k = 5 : TransferFcn  Numerator=[m_G(5)*T 0]  Denominator=[T n(5)]
  k = 6 : TransferFcn  Numerator=[m_G(6)*T 0]  Denominator=[T n(6)]
  G : Outport
  wires:
  Sum/1 -> G/1
  F + P_1/1 -> k = 4/1, k = 6/1, k = 5/1, k = 1/1, Sum/1, k = 2/1, k = 3/1
  k = 3/1 -> Sum/4
  k = 1/1 -> Sum/2
  k = 2/1 -> Sum/3
  k = 4/1 -> Sum/5
  k = 5/1 -> Sum/6
  k = 6/1 -> Sum/7

== system usask_tlm_lib/Tapered Elastic TLM Q1Q2/G_2 ==
  note: Equation (17) from ven der Buhs et al. 2017
  F + P_2 : Inport
  Sum : Sum  Inputs=+------
  k = 1 : TransferFcn  Numerator=[m_G(1)*T 0]  Denominator=[T n(1)]
  k = 2 : TransferFcn  Numerator=[m_G(2)*T 0]  Denominator=[T n(2)]
  k = 3 : TransferFcn  Numerator=[m_G(3)*T 0]  Denominator=[T n(3)]
  k = 4 : TransferFcn  Numerator=[m_G(4)*T 0]  Denominator=[T n(4)]
  k = 5 : TransferFcn  Numerator=[m_G(5)*T 0]  Denominator=[T n(5)]
  k = 6 : TransferFcn  Numerator=[m_G(6)*T 0]  Denominator=[T n(6)]
  G : Outport
  wires:
  Sum/1 -> G/1
  F + P_2/1 -> k = 4/1, k = 6/1, k = 5/1, k = 1/1, Sum/1, k = 2/1, k = 3/1
  k = 3/1 -> Sum/4
  k = 1/1 -> Sum/2
  k = 2/1 -> Sum/3
  k = 4/1 -> Sum/5
  k = 5/1 -> Sum/6
  k = 6/1 -> Sum/7

== system usask_tlm_lib/Tapered TLM P1P2/  Delay_2  ==
  G : Inport
  Transport Delay : TransportDelay  DelayTime=T_prime
  delay : Outport
  wires:
  Transport Delay/1 -> delay/1
  G/1 -> Transport Delay/1

== system usask_tlm_lib/Tapered TLM P1P2/Delay_1  ==
  G : Inport
  Transport Delay : TransportDelay  DelayTime=T_prime
  delay : Outport
  wires:
  Transport Delay/1 -> delay/1
  G/1 -> Transport Delay/1

== system usask_tlm_lib/Tapered TLM P1P2/E_1 ==
  note: Equation (14) from ven der Buhs et al. 2017
  Q_1 : Inport
  Gain : Gain  Gain=Z_c
  Sum : Sum  Inputs=++++++
  k = 1 : TransferFcn  Numerator=[m_E(1)]  Denominator=[T n(1)]
  k = 2 : TransferFcn  Numerator=[m_E(2)]  Denominator=[T n(2)]
  k = 3 : TransferFcn  Numerator=[m_E(3)]  Denominator=[T n(3)]
  k = 4 : TransferFcn  Numerator=[m_E(4)]  Denominator=[T n(4)]
  k = 5 : TransferFcn  Numerator=[m_E(5)]  Denominator=[T n(5)]
  k = 6 : TransferFcn  Numerator=[m_E(6)]  Denominator=[T n(6)]
  E : Outport
  wires:
  Q_1/1 -> k = 4/1, k = 5/1, k = 6/1, k = 3/1, k = 1/1, k = 2/1
  k = 6/1 -> Sum/6
  k = 5/1 -> Sum/5
  k = 4/1 -> Sum/4
  k = 3/1 -> Sum/3
  k = 2/1 -> Sum/2
  k = 1/1 -> Sum/1
  Sum/1 -> Gain/1
  Gain/1 -> E/1

== system usask_tlm_lib/Tapered TLM P1P2/E_2 ==
  note: Equation (14) from ven der Buhs et al. 2017
  Q_2 : Inport
  Gain : Gain  Gain=Z_c
  Sum : Sum  Inputs=++++++
  k = 1 : TransferFcn  Numerator=[m_E(1)]  Denominator=[T n(1)]
  k = 2 : TransferFcn  Numerator=[m_E(2)]  Denominator=[T n(2)]
  k = 3 : TransferFcn  Numerator=[m_E(3)]  Denominator=[T n(3)]
  k = 4 : TransferFcn  Numerator=[m_E(4)]  Denominator=[T n(4)]
  k = 5 : TransferFcn  Numerator=[m_E(5)]  Denominator=[T n(5)]
  k = 6 : TransferFcn  Numerator=[m_E(6)]  Denominator=[T n(6)]
  E : Outport
  wires:
  Q_2/1 -> k = 4/1, k = 5/1, k = 6/1, k = 3/1, k = 1/1, k = 2/1
  k = 6/1 -> Sum/6
  k = 5/1 -> Sum/5
  k = 4/1 -> Sum/4
  k = 3/1 -> Sum/3
  k = 2/1 -> Sum/2
  k = 1/1 -> Sum/1
  Sum/1 -> Gain/1
  Gain/1 -> E/1

== system usask_tlm_lib/Tapered TLM P1P2/F_1 ==
  note: Equation (15) from ven der Buhs et al. 2017
  Q_1 : Inport
  E : Inport  Port=2
  Gain : Gain  Gain=b
  Gain1 : Gain  Gain=Z_c
  Sum : Sum
  Out1 : Outport
  wires:
  E/1 -> Gain/1
  Q_1/1 -> Gain1/1
  Sum/1 -> Out1/1
  Gain1/1 -> Sum/1
  Gain/1 -> Sum/2

== system usask_tlm_lib/Tapered TLM P1P2/F_2 ==
  note: Equation (15) from ven der Buhs et al. 2017
  E : Inport
  Q_2 : Inport  Port=2
  Gain : Gain  Gain=b
  Gain1 : Gain  Gain=Z_c
  Sum : Sum
  F : Outport
  wires:
  Gain/1 -> Sum/2
  Gain1/1 -> Sum/1
  Sum/1 -> F/1
  Q_2/1 -> Gain1/1
  E/1 -> Gain/1

== system usask_tlm_lib/Tapered TLM P1P2/G_1 ==
  note: Equation (17) from ven der Buhs et al. 2017
  F + P_1 : Inport
  Sum : Sum  Inputs=+------
  k = 1 : TransferFcn  Numerator=[m_G(1)*T 0]  Denominator=[T n(1)]
  k = 2 : TransferFcn  Numerator=[m_G(2)*T 0]  Denominator=[T n(2)]
  k = 3 : TransferFcn  Numerator=[m_G(3)*T 0]  Denominator=[T n(3)]
  k = 4 : TransferFcn  Numerator=[m_G(4)*T 0]  Denominator=[T n(4)]
  k = 5 : TransferFcn  Numerator=[m_G(5)*T 0]  Denominator=[T n(5)]
  k = 6 : TransferFcn  Numerator=[m_G(6)*T 0]  Denominator=[T n(6)]
  G : Outport
  wires:
  k = 6/1 -> Sum/7
  k = 5/1 -> Sum/6
  k = 4/1 -> Sum/5
  k = 2/1 -> Sum/3
  k = 1/1 -> Sum/2
  k = 3/1 -> Sum/4
  F + P_1/1 -> k = 3/1, k = 2/1, Sum/1, k = 1/1, k = 5/1, k = 6/1, k = 4/1
  Sum/1 -> G/1

== system usask_tlm_lib/Tapered TLM P1P2/G_2 ==
  note: Equation (17) from ven der Buhs et al. 2017
  F + P_2 : Inport
  Sum : Sum  Inputs=+------
  k = 1 : TransferFcn  Numerator=[m_G(1)*T 0]  Denominator=[T n(1)]
  k = 2 : TransferFcn  Numerator=[m_G(2)*T 0]  Denominator=[T n(2)]
  k = 3 : TransferFcn  Numerator=[m_G(3)*T 0]  Denominator=[T n(3)]
  k = 4 : TransferFcn  Numerator=[m_G(4)*T 0]  Denominator=[T n(4)]
  k = 5 : TransferFcn  Numerator=[m_G(5)*T 0]  Denominator=[T n(5)]
  k = 6 : TransferFcn  Numerator=[m_G(6)*T 0]  Denominator=[T n(6)]
  G : Outport
  wires:
  k = 6/1 -> Sum/7
  k = 5/1 -> Sum/6
  k = 4/1 -> Sum/5
  k = 2/1 -> Sum/3
  k = 1/1 -> Sum/2
  k = 3/1 -> Sum/4
  F + P_2/1 -> k = 3/1, k = 2/1, Sum/1, k = 1/1, k = 5/1, k = 6/1, k = 4/1
  Sum/1 -> G/1

== system usask_tlm_lib/Tapered TLM P1Q2/  Delay_2  ==
  G : Inport
  Transport Delay : TransportDelay  DelayTime=T_prime
  delay : Outport
  wires:
  Transport Delay/1 -> delay/1
  G/1 -> Transport Delay/1

== system usask_tlm_lib/Tapered TLM P1Q2/Delay_1  ==
  G : Inport
  Transport Delay : TransportDelay  DelayTime=T_prime
  delay : Outport
  wires:
  Transport Delay/1 -> delay/1
  G/1 -> Transport Delay/1

== system usask_tlm_lib/Tapered TLM P1Q2/E_1 ==
  note: Equation (14) from ven der Buhs et al. 2017
  Q_1 : Inport
  Gain : Gain  Gain=Z_c
  Sum : Sum  Inputs=++++++
  k = 1 : TransferFcn  Numerator=[m_E(1)]  Denominator=[T n(1)]
  k = 2 : TransferFcn  Numerator=[m_E(2)]  Denominator=[T n(2)]
  k = 3 : TransferFcn  Numerator=[m_E(3)]  Denominator=[T n(3)]
  k = 4 : TransferFcn  Numerator=[m_E(4)]  Denominator=[T n(4)]
  k = 5 : TransferFcn  Numerator=[m_E(5)]  Denominator=[T n(5)]
  k = 6 : TransferFcn  Numerator=[m_E(6)]  Denominator=[T n(6)]
  E : Outport
  wires:
  Q_1/1 -> k = 4/1, k = 5/1, k = 6/1, k = 3/1, k = 1/1, k = 2/1
  k = 6/1 -> Sum/6
  k = 5/1 -> Sum/5
  k = 4/1 -> Sum/4
  k = 3/1 -> Sum/3
  k = 2/1 -> Sum/2
  k = 1/1 -> Sum/1
  Sum/1 -> Gain/1
  Gain/1 -> E/1

== system usask_tlm_lib/Tapered TLM P1Q2/E_2 ==
  note: Equation (14) from ven der Buhs et al. 2017
  Q_2 : Inport
  Gain : Gain  Gain=Z_c
  Sum : Sum  Inputs=++++++
  k = 1 : TransferFcn  Numerator=[m_E(1)]  Denominator=[T n(1)]
  k = 2 : TransferFcn  Numerator=[m_E(2)]  Denominator=[T n(2)]
  k = 3 : TransferFcn  Numerator=[m_E(3)]  Denominator=[T n(3)]
  k = 4 : TransferFcn  Numerator=[m_E(4)]  Denominator=[T n(4)]
  k = 5 : TransferFcn  Numerator=[m_E(5)]  Denominator=[T n(5)]
  k = 6 : TransferFcn  Numerator=[m_E(6)]  Denominator=[T n(6)]
  E : Outport
  wires:
  Q_2/1 -> k = 4/1, k = 5/1, k = 6/1, k = 3/1, k = 1/1, k = 2/1
  k = 6/1 -> Sum/6
  k = 5/1 -> Sum/5
  k = 4/1 -> Sum/4
  k = 3/1 -> Sum/3
  k = 2/1 -> Sum/2
  k = 1/1 -> Sum/1
  Sum/1 -> Gain/1
  Gain/1 -> E/1

== system usask_tlm_lib/Tapered TLM P1Q2/F_1 ==
  note: Equation (15) from ven der Buhs et al. 2017
  Q_1 : Inport
  E : Inport  Port=2
  Gain : Gain  Gain=b
  Gain1 : Gain  Gain=Z_c
  Sum : Sum
  F : Outport
  wires:
  E/1 -> Gain/1
  Q_1/1 -> Gain1/1
  Sum/1 -> F/1
  Gain1/1 -> Sum/1
  Gain/1 -> Sum/2

== system usask_tlm_lib/Tapered TLM P1Q2/F_2 ==
  note: Equation (15) from ven der Buhs et al. 2017
  E : Inport
  Q_2 : Inport  Port=2
  Gain : Gain  Gain=b
  Gain1 : Gain  Gain=Z_c
  Sum : Sum
  Out1 : Outport
  wires:
  Gain/1 -> Sum/2
  Gain1/1 -> Sum/1
  Sum/1 -> Out1/1
  Q_2/1 -> Gain1/1
  E/1 -> Gain/1

== system usask_tlm_lib/Tapered TLM P1Q2/G_1 ==
  note: Equation (17) from ven der Buhs et al. 2017
  F + P_1 : Inport
  Sum : Sum  Inputs=+------
  k = 1 : TransferFcn  Numerator=[m_G(1)*T 0]  Denominator=[T n(1)]
  k = 2 : TransferFcn  Numerator=[m_G(2)*T 0]  Denominator=[T n(2)]
  k = 3 : TransferFcn  Numerator=[m_G(3)*T 0]  Denominator=[T n(3)]
  k = 4 : TransferFcn  Numerator=[m_G(4)*T 0]  Denominator=[T n(4)]
  k = 5 : TransferFcn  Numerator=[m_G(5)*T 0]  Denominator=[T n(5)]
  k = 6 : TransferFcn  Numerator=[m_G(6)*T 0]  Denominator=[T n(6)]
  G : Outport
  wires:
  k = 6/1 -> Sum/7
  k = 5/1 -> Sum/6
  k = 4/1 -> Sum/5
  k = 2/1 -> Sum/3
  k = 1/1 -> Sum/2
  k = 3/1 -> Sum/4
  F + P_1/1 -> k = 3/1, k = 2/1, Sum/1, k = 1/1, k = 5/1, k = 6/1, k = 4/1
  Sum/1 -> G/1

== system usask_tlm_lib/Tapered TLM P1Q2/G_2 ==
  note: Equation (17) from ven der Buhs et al. 2017
  F + P_2 : Inport
  Sum : Sum  Inputs=+------
  k = 1 : TransferFcn  Numerator=[m_G(1)*T 0]  Denominator=[T n(1)]
  k = 2 : TransferFcn  Numerator=[m_G(2)*T 0]  Denominator=[T n(2)]
  k = 3 : TransferFcn  Numerator=[m_G(3)*T 0]  Denominator=[T n(3)]
  k = 4 : TransferFcn  Numerator=[m_G(4)*T 0]  Denominator=[T n(4)]
  k = 5 : TransferFcn  Numerator=[m_G(5)*T 0]  Denominator=[T n(5)]
  k = 6 : TransferFcn  Numerator=[m_G(6)*T 0]  Denominator=[T n(6)]
  G : Outport
  wires:
  k = 6/1 -> Sum/7
  k = 5/1 -> Sum/6
  k = 4/1 -> Sum/5
  k = 2/1 -> Sum/3
  k = 1/1 -> Sum/2
  k = 3/1 -> Sum/4
  F + P_2/1 -> k = 3/1, k = 2/1, Sum/1, k = 1/1, k = 5/1, k = 6/1, k = 4/1
  Sum/1 -> G/1

== system usask_tlm_lib/Tapered TLM Q1P2/  Delay_2  ==
  G : Inport
  Transport Delay : TransportDelay  DelayTime=T_prime
  delay : Outport
  wires:
  Transport Delay/1 -> delay/1
  G/1 -> Transport Delay/1

== system usask_tlm_lib/Tapered TLM Q1P2/Delay_1  ==
  G : Inport
  Transport Delay : TransportDelay  DelayTime=T_prime
  delay : Outport
  wires:
  Transport Delay/1 -> delay/1
  G/1 -> Transport Delay/1

== system usask_tlm_lib/Tapered TLM Q1P2/E_1 ==
  note: Equation (14) from ven der Buhs et al. 2017
  Q_1 : Inport
  Gain : Gain  Gain=Z_c
  Sum : Sum  Inputs=++++++
  k = 1 : TransferFcn  Numerator=[m_E(1)]  Denominator=[T n(1)]
  k = 2 : TransferFcn  Numerator=[m_E(2)]  Denominator=[T n(2)]
  k = 3 : TransferFcn  Numerator=[m_E(3)]  Denominator=[T n(3)]
  k = 4 : TransferFcn  Numerator=[m_E(4)]  Denominator=[T n(4)]
  k = 5 : TransferFcn  Numerator=[m_E(5)]  Denominator=[T n(5)]
  k = 6 : TransferFcn  Numerator=[m_E(6)]  Denominator=[T n(6)]
  E : Outport
  wires:
  Q_1/1 -> k = 4/1, k = 5/1, k = 6/1, k = 3/1, k = 1/1, k = 2/1
  k = 6/1 -> Sum/6
  k = 5/1 -> Sum/5
  k = 4/1 -> Sum/4
  k = 3/1 -> Sum/3
  k = 2/1 -> Sum/2
  k = 1/1 -> Sum/1
  Sum/1 -> Gain/1
  Gain/1 -> E/1

== system usask_tlm_lib/Tapered TLM Q1P2/E_2 ==
  note: Equation (14) from ven der Buhs et al. 2017
  Q_2 : Inport
  Gain : Gain  Gain=Z_c
  Sum : Sum  Inputs=++++++
  k = 1 : TransferFcn  Numerator=[m_E(1)]  Denominator=[T n(1)]
  k = 2 : TransferFcn  Numerator=[m_E(2)]  Denominator=[T n(2)]
  k = 3 : TransferFcn  Numerator=[m_E(3)]  Denominator=[T n(3)]
  k = 4 : TransferFcn  Numerator=[m_E(4)]  Denominator=[T n(4)]
  k = 5 : TransferFcn  Numerator=[m_E(5)]  Denominator=[T n(5)]
  k = 6 : TransferFcn  Numerator=[m_E(6)]  Denominator=[T n(6)]
  E : Outport
  wires:
  Q_2/1 -> k = 4/1, k = 5/1, k = 6/1, k = 3/1, k = 1/1, k = 2/1
  k = 6/1 -> Sum/6
  k = 5/1 -> Sum/5
  k = 4/1 -> Sum/4
  k = 3/1 -> Sum/3
  k = 2/1 -> Sum/2
  k = 1/1 -> Sum/1
  Sum/1 -> Gain/1
  Gain/1 -> E/1

== system usask_tlm_lib/Tapered TLM Q1P2/F_1 ==
  note: Equation (15) from ven der Buhs et al. 2017
  Q_1 : Inport
  E : Inport  Port=2
  Gain : Gain  Gain=b
  Gain1 : Gain  Gain=Z_c
  Sum : Sum
  F : Outport
  wires:
  E/1 -> Gain/1
  Q_1/1 -> Gain1/1
  Sum/1 -> F/1
  Gain1/1 -> Sum/1
  Gain/1 -> Sum/2

== system usask_tlm_lib/Tapered TLM Q1P2/F_2 ==
  note: Equation (15) from ven der Buhs et al. 2017
  E : Inport
  Q_2 : Inport  Port=2
  Gain : Gain  Gain=b
  Gain1 : Gain  Gain=Z_c
  Sum : Sum
  Out1 : Outport
  wires:
  Gain/1 -> Sum/2
  Gain1/1 -> Sum/1
  Sum/1 -> Out1/1
  Q_2/1 -> Gain1/1
  E/1 -> Gain/1
